simulink model "FOC_Motor"  (R2023b)
settings: Solver=FixedStepDiscrete  StartTime=0.0  StopTime=10  FixedStep=0.0001  RelTol=1e-3
undefined symbols (not defined in the file): Cos_Table, Sin_BreakPoint, Sin_Table
libraries: simulink x3
settings Model: DataDictionary=EHB_data.sldd  Creator=dell  LastModifiedBy=LQY
settings SolverCC: AlgebraicLoopSolver=TrustRegion  PositivePriorityOrder=on  AutoInsertRateTranBlk=on
settings DataIOCC: LimitDataPoints=on  SaveFormat=Structure  SignalLoggingSaveFormat=ModelDataLogs  ReturnWorkspaceOutputs=off
settings OptimizationCC: DefaultParameterBehavior=Inlined  UseDivisionForNetSlopeComputation=on  GainParamInheritBuiltInType=on  UseFloatMulNetSlope=on  InlineInvariantSignals=on  PassReuseOutputArgsAs=Individual arguments  ExpressionDepthLimit=2147483647  ZeroExternalMemoryAtStartup=off  ZeroInternalMemoryAtStartup=off  NoFixptDivByZeroProtection=on  EfficientFloat2IntCast=on  LifeSpan=1  MaxStackSize=64  EfficientTunableParamExpr=on
settings DebuggingCC: CheckSSInitialOutputMsg=off  UnderspecifiedInitializationDetection=Classic  MergeDetectMultiDrivingBlocksExec=none  SolverPrmCheckMsg=warning  ParameterOverflowMsg=none  ParameterPrecisionLossMsg=none  FcnCallInpInsideContextMsg=warning  UnconnectedInputMsg=warning  UnconnectedOutputMsg=warning  UnconnectedLineMsg=warning  AssertControl=EnableAll  StateNameClashWarn=warning  SFUnexpectedBacktrackingDiag=warning  SFNoUnconditionalDefaultTransitionDiag=warning  SFExecutionAtInitializationDiag=none  ArithmeticOperatorsInVariantConditions=warning
settings HardwareCC: ProdBitPerPointer=32  ProdBitPerSizeT=32  ProdBitPerPtrDiffT=32  ProdLargestAtomicInteger=Long  ProdLargestAtomicFloat=Double  ProdWordSize=32  ProdLongLongMode=on  ProdHWDeviceType=NXP->Cortex-M0/M0+  TargetBitPerPointer=64  TargetBitPerSizeT=64  TargetBitPerPtrDiffT=64  TargetLargestAtomicInteger=Integer  TargetLongLongMode=on  TargetIntDivRoundTo=Zero  TargetEndianess=LittleEndian  TargetWordSize=64  TargetHWDeviceType=MATLAB Host  ProdEqTarget=off
settings ModelReferenceCC: UpdateModelReferenceTargets=IfOutOfDate  EnableRefExpFcnMdlSchedulingChecks=on  PropagateSignalLabelsOutOfModel=off
settings SFSimCC: SimUseLocalCustomCode=off  MATLABDynamicMemAlloc=off  CustomCodeUndefinedFunction=UseInterfaceOnly
settings SFSimCC: SimCustomHeaderCode=|
  | #define MCU_IDLE_ST     0
  | #define MCU_INIT_ST     1
  | #define MCU_START_ST    2
  | #define MCU_RUN_ST      3
  | #define MCU_FAULT_ST    4
  | #define MCU_WAIT_ST     5
  | 
  | // MCU_IDLE_ST = 0;
  | // MCU_INIT_ST = 1;
  | // MCU_START_ST = 2;
  | // MCU_RUN_ST = 3;
  | // MCU_FAULT_ST = 4;
  | // MCU_WAIT_ST = 5;
settings RTWCC: Description=Embedded Coder  SystemTargetFile=ert.tlc  GenCodeOnly=on  TemplateMakefile=ert_default_tmf  RTWUseLocalCustomCode=off  RTWUseSimCustomCode=on  IncludeHyperlinkInReport=on
settings RTWCC: CustomHeaderCode=|
  | #define MCU_IDLE_ST     0
  | #define MCU_INIT_ST     1
  | #define MCU_START_ST    2
  | #define MCU_RUN_ST      3
  | #define MCU_FAULT_ST    4
  | #define MCU_WAIT_ST     5
  | 
  | // MCU_IDLE_ST = 0;
  | // MCU_INIT_ST = 1;
  | // MCU_START_ST = 2;
  | // MCU_RUN_ST = 3;
  | // MCU_FAULT_ST = 4;
  | // MCU_WAIT_ST = 5;
settings CodeAppCC: ForceParamTrailComments=on  IgnoreCustomStorageClasses=off  SimulinkDataObjDesc=on  CustomSymbolStrGlobalVar=rt$N$M  CustomSymbolStrType=$N$M  CustomSymbolStrFcn=$N$M$F  CustomSymbolStrMacro=$N$M  InsertBlockDesc=on  InternalIdentifier=Classic
settings ERTTargetCC: MultiwordLength=2048  IncludeMdlTerminateFcn=off  CombineSignalStateStructs=on  IncludeFileDelimiter=UseQuote  SupportAbsoluteTime=off  SupportComplex=off  SupportNonInlinedSFcns=on  InlinedParameterPlacement=NonHierarchical  ERTCustomFileTemplate=example_file_process.tlc  GlobalDataDefinition=InSeparateSourceFile  DataDefinitionFile=EHB_MOTOR_data.c  GlobalDataReference=InSeparateHeaderFile  ERTFilePackagingFormat=CompactWithDataFile  DataReferenceFile=EHB_MOTOR.h  ConvertIfToSwitch=off  SuppressUnreachableDefaultCases=off  IndentStyle=Allman  IndentSize=4  MemSecPackage=mpt
settings ConfigComp: CovMetricSettings=dw  CovSaveCumulativeToWorkspaceVar=on  CovSaveSingleToWorkspaceVar=on  CovExternalEMLEnable=off  CovSFcnEnable=off
settings SimscapeCC: SimscapeNormalizeSystem=off
settings ConfigurationSet: Description=SimMechanics 2G

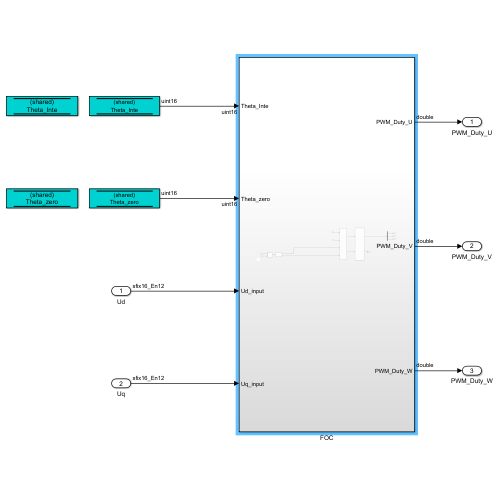
[thumbnail: Simulink's stored preview of the top-level diagram]
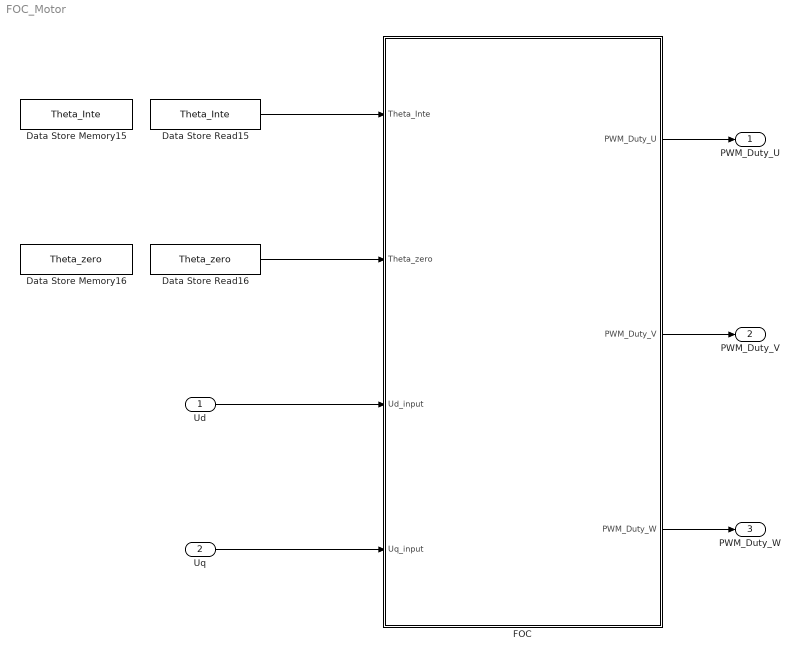
== system FOC_Motor ==
  Ud : Inport  OutDataTypeStr=fixdt(1,16,12)
  Uq : Inport  Port=2  OutDataTypeStr=fixdt(1,16,12)
  Data Store Memory15 : DataStoreMemory  DataStoreName=Theta_Inte  ReadBeforeWriteMsg=warning  WriteAfterWriteMsg=warning  WriteAfterReadMsg=warning  ShareAcrossModelInstances=on  ShowAdditionalParam=off  OutDataTypeStr=uint16
  Data Store Memory16 : DataStoreMemory  DataStoreName=Theta_zero  ReadBeforeWriteMsg=warning  WriteAfterWriteMsg=warning  WriteAfterReadMsg=warning  ShareAcrossModelInstances=on  ShowAdditionalParam=off  OutDataTypeStr=uint16
  Data Store Read15 : DataStoreRead  DataStoreName=Theta_Inte  DataStoreElements=Theta_Inte  IndexOptions=Index vector (dialog)  Indices=1  OutputSizes=1
  Data Store Read16 : DataStoreRead  DataStoreName=Theta_zero  DataStoreElements=Theta_zero  IndexOptions=Index vector (dialog)  Indices=1  OutputSizes=1
  FOC : Subsystem
  PWM_Duty_U : Outport  VectorParamsAs1DForOutWhenUnconnected=off
  PWM_Duty_V : Outport  Port=2  VectorParamsAs1DForOutWhenUnconnected=off
  PWM_Duty_W : Outport  Port=3  VectorParamsAs1DForOutWhenUnconnected=off
  wires:
  Data Store Read15/1 -> FOC/1(Theta_Inte)
  FOC/2(PWM_Duty_V) -> PWM_Duty_V/1
  FOC/1(PWM_Duty_U) -> PWM_Duty_U/1
  FOC/3(PWM_Duty_W) -> PWM_Duty_W/1
  Data Store Read16/1 -> FOC/2(Theta_zero)
  Ud/1 -> FOC/3(Ud_input)
  Uq/1 -> FOC/4(Uq_input)

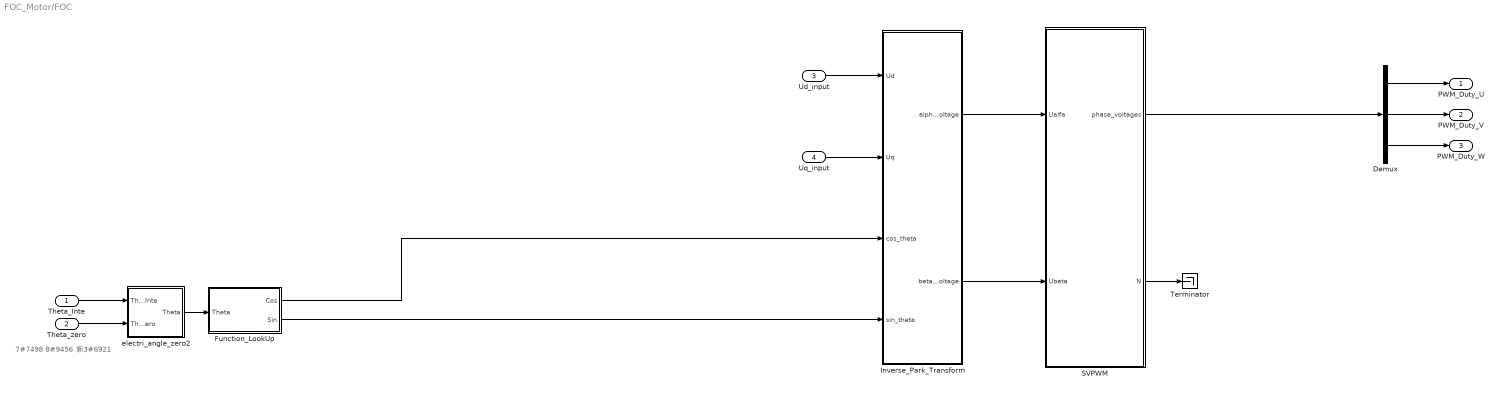
== system FOC_Motor/FOC ==
  note: 7#7498
      | 8#9456
      | 新3#6921
  Theta_Inte : Inport  OutDataTypeStr=uint16
  Theta_zero : Inport  Port=2  OutDataTypeStr=uint16
  Ud_input : Inport  Port=3
  Uq_input : Inport  Port=4
  Demux : Demux  Outputs=3
  Function_LookUp : Subsystem
  Inverse_Park_Transform : Subsystem
  SVPWM : Subsystem
  Terminator : Terminator
  electri_angle_zero2 : Subsystem
  PWM_Duty_U : Outport  VectorParamsAs1DForOutWhenUnconnected=off
  PWM_Duty_V : Outport  Port=2  VectorParamsAs1DForOutWhenUnconnected=off
  PWM_Duty_W : Outport  Port=3  VectorParamsAs1DForOutWhenUnconnected=off
  wires:
  Inverse_Park_Transform/2(beta_voltage) -> SVPWM/2(Ubeta)
  Demux/1 -> PWM_Duty_U/1
  Theta_zero/1 -> electri_angle_zero2/2(Theta_zero)
  Uq_input/1 -> Inverse_Park_Transform/2(Uq)
  Theta_Inte/1 -> electri_angle_zero2/1(Theta_Inte)
  Inverse_Park_Transform/1(alpha_voltage) -> SVPWM/1(Ualfa)
  Ud_input/1 -> Inverse_Park_Transform/1(Ud)
  SVPWM/1(phase_voltages) -> Demux/1
  Demux/3 -> PWM_Duty_W/1
  Demux/2 -> PWM_Duty_V/1
  Function_LookUp/1(Cos) -> Inverse_Park_Transform/3(cos_theta)
  Function_LookUp/2(Sin) -> Inverse_Park_Transform/4(sin_theta)
  electri_angle_zero2/1(Theta) -> Function_LookUp/1(Theta)
  SVPWM/2(N) -> Terminator/1

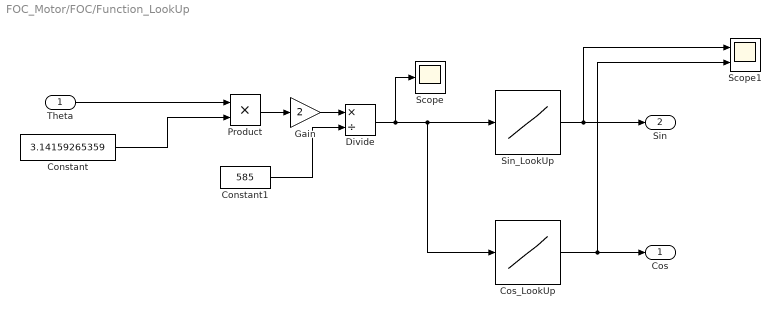
== system FOC_Motor/FOC/Function_LookUp ==
  Theta : Inport
  Constant : Constant  Value=3.14159265359
  Constant1 : Constant  Value=585
  Cos_LookUp : Lookup_n-D  NumberOfTableDimensions=1  BreakpointsForDimension1=Sin_BreakPoint  BreakpointsForDimension3=[5, 7]  BreakpointsForDimension1DataTypeStr=Inherit: Inherit from 'Breakpoint data'  Table=Cos_Table  TableDataTypeStr=Inherit: Inherit from 'Table data'  ExtrapMethod=Clip  InternalRulePriority=Speed  OutDataTypeStr=Inherit: Inherit from 'Table data'  RndMeth=Simplest  InputSameDT=off
  Divide : Product  Inputs=*/
  Gain : Gain  Gain=2
  Product : Product
  Scope : Scope
  Scope1 : Scope  NumInputPorts=2
  Sin_LookUp : Lookup_n-D  NumberOfTableDimensions=1  BreakpointsForDimension1=Sin_BreakPoint  BreakpointsForDimension3=[5, 7]  BreakpointsForDimension1DataTypeStr=Inherit: Inherit from 'Breakpoint data'  Table=Sin_Table  TableDataTypeStr=Inherit: Inherit from 'Table data'  ExtrapMethod=Clip  InternalRulePriority=Speed  OutDataTypeStr=Inherit: Inherit from 'Table data'  RndMeth=Simplest  InputSameDT=off
  Cos : Outport  VectorParamsAs1DForOutWhenUnconnected=off
  Sin : Outport  Port=2  VectorParamsAs1DForOutWhenUnconnected=off
  wires:
  Divide/1 -> Scope/1, Cos_LookUp/1, Sin_LookUp/1
  Theta/1 -> Product/1
  Cos_LookUp/1 -> Scope1/2, Cos/1
  Constant/1 -> Product/2
  Product/1 -> Gain/1
  Constant1/1 -> Divide/2
  Gain/1 -> Divide/1
  Sin_LookUp/1 -> Scope1/1, Sin/1

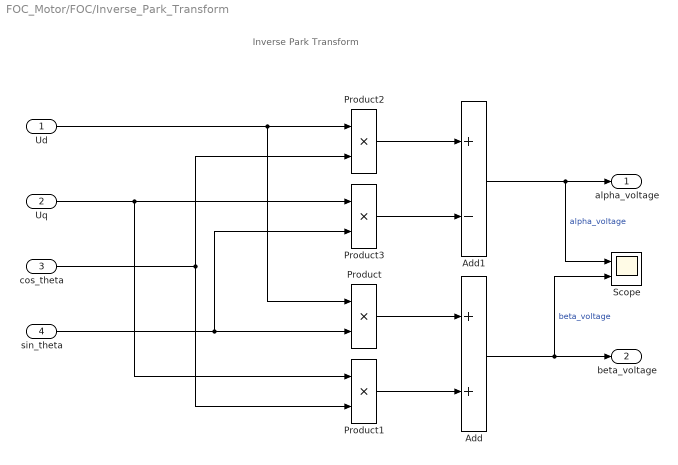
== system FOC_Motor/FOC/Inverse_Park_Transform ==
  note: Inverse Park Transform
  Ud : Inport
  Uq : Inport  Port=2
  cos_theta : Inport  Port=3
  sin_theta : Inport  Port=4
  Add : Sum  OutDataTypeStr=fixdt(1,16,12)
  Add1 : Sum  Inputs=+-  OutDataTypeStr=fixdt(1,16,12)
  Product{,1..3} (4 alike) : Product  OutDataTypeStr=fixdt(1,16,12)  RndMeth=Zero
  Scope : Scope  NumInputPorts=2
  alpha_voltage : Outport  VectorParamsAs1DForOutWhenUnconnected=off
  beta_voltage : Outport  Port=2  VectorParamsAs1DForOutWhenUnconnected=off
  wires:
  Product/1 -> Add/1
  Product1/1 -> Add/2
  Add/1 -> Scope/2, beta_voltage/1  "beta_voltage"
  Product2/1 -> Add1/1
  Product3/1 -> Add1/2
  Add1/1 -> Scope/1, alpha_voltage/1  "alpha_voltage"
  Ud/1 -> Product/1, Product2/1
  sin_theta/1 -> Product/2, Product3/2
  cos_theta/1 -> Product1/2, Product2/2
  Uq/1 -> Product1/1, Product3/1

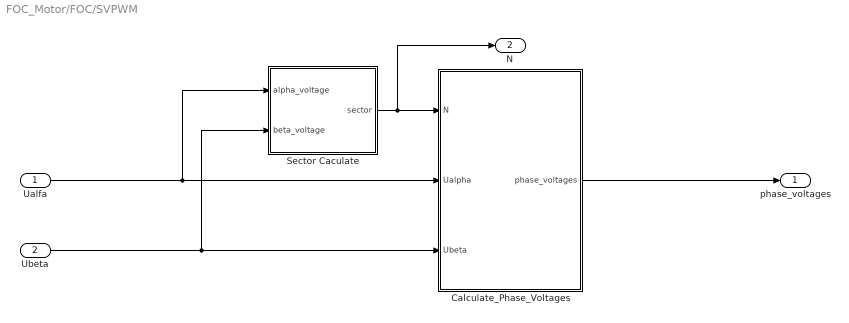
== system FOC_Motor/FOC/SVPWM ==
  Ualfa : Inport  OutDataTypeStr=fixdt(1,16,12)
  Ubeta : Inport  Port=2
  Calculate_Phase_Voltages : Subsystem
  Sector Caculate : Subsystem
  phase_voltages : Outport  VectorParamsAs1DForOutWhenUnconnected=off
  N : Outport  Port=2  VectorParamsAs1DForOutWhenUnconnected=off
  wires:
  Ualfa/1 -> Sector Caculate/1(alpha_voltage), Calculate_Phase_Voltages/2(Ualpha)
  Ubeta/1 -> Calculate_Phase_Voltages/3(Ubeta), Sector Caculate/2(beta_voltage)
  Calculate_Phase_Voltages/1(phase_voltages) -> phase_voltages/1
  Sector Caculate/1(sector) -> N/1, Calculate_Phase_Voltages/1(N)

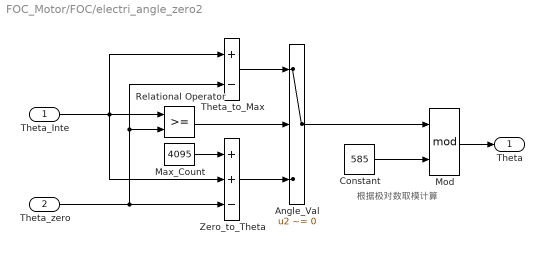
== system FOC_Motor/FOC/electri_angle_zero2 ==
  note: 根据极对数取模计算
  Theta_Inte : Inport
  Theta_zero : Inport  Port=2  OutDataTypeStr=uint16
  Angle_Val : Switch  Criteria=u2 ~= 0  Threshold=3032  OutDataTypeStr=uint16  SaturateOnIntegerOverflow=off  InputSameDT=off
  Constant : Constant  Value=585  OutDataTypeStr=uint16
  Max_Count : Constant  Value=4095  OutDataTypeStr=uint16
  Mod : Math  Operator=mod  SignedPower=on
  Relational Operator : RelationalOperator  OutDataTypeStr=boolean  InputSameDT=off
  Theta_to_Max : Sum  Inputs=+-  OutDataTypeStr=uint16
  Zero_to_Theta : Sum  Inputs=++-  OutDataTypeStr=uint16
  Theta : Outport  VectorParamsAs1DForOutWhenUnconnected=off
  wires:
  Max_Count/1 -> Zero_to_Theta/1
  Theta_zero/1 -> Zero_to_Theta/3, Theta_to_Max/2, Relational Operator/2
  Theta_Inte/1 -> Zero_to_Theta/2, Theta_to_Max/1, Relational Operator/1
  Zero_to_Theta/1 -> Angle_Val/3
  Angle_Val/1 -> Mod/1
  Theta_to_Max/1 -> Angle_Val/1
  Relational Operator/1 -> Angle_Val/2
  Mod/1 -> Theta/1
  Constant/1 -> Mod/2

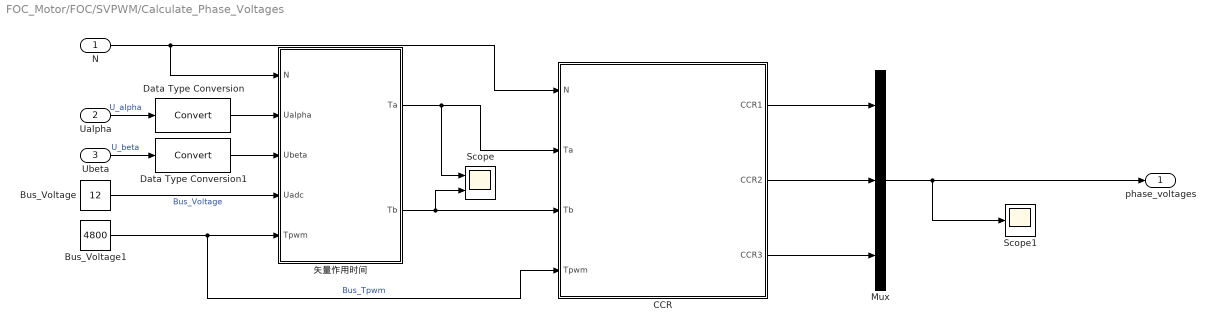
== system FOC_Motor/FOC/SVPWM/Calculate_Phase_Voltages ==
  N : Inport  OutDataTypeStr=uint8
  Ualpha : Inport  Port=2
  Ubeta : Inport  Port=3
  Bus_Voltage : Constant  Value=12  OutDataTypeStr=double
  Bus_Voltage1 : Constant  Value=4800  OutDataTypeStr=double
  CCR : MATLAB Function  TreatAsAtomicUnit=on
  Data Type Conversion : DataTypeConversion  SaturateOnIntegerOverflow=off  RndMeth=Floor
  Data Type Conversion1 : DataTypeConversion  SaturateOnIntegerOverflow=off  RndMeth=Floor
  Mux : Mux  Inputs=3
  Scope : Scope  NumInputPorts=2
  Scope1 : Scope
  矢量作用时间 : MATLAB Function  TreatAsAtomicUnit=on
  phase_voltages : Outport  VectorParamsAs1DForOutWhenUnconnected=off
  wires:
  Ualpha/1 -> Data Type Conversion/1  "U_alpha"
  Ubeta/1 -> Data Type Conversion1/1  "U_beta"
  Bus_Voltage/1 -> 矢量作用时间/4(Uadc)  "Bus_Voltage"
  N/1 -> 矢量作用时间/1(N), CCR/1(N)
  Bus_Voltage1/1 -> CCR/4(Tpwm), 矢量作用时间/5(Tpwm)  "Bus_Tpwm"
  矢量作用时间/1(Ta) -> Scope/1, CCR/2(Ta)
  矢量作用时间/2(Tb) -> Scope/2, CCR/3(Tb)
  CCR/1(CCR1) -> Mux/1
  CCR/2(CCR2) -> Mux/2
  CCR/3(CCR3) -> Mux/3
  Mux/1 -> Scope1/1, phase_voltages/1
  Data Type Conversion/1 -> 矢量作用时间/2(Ualpha)
  Data Type Conversion1/1 -> 矢量作用时间/3(Ubeta)

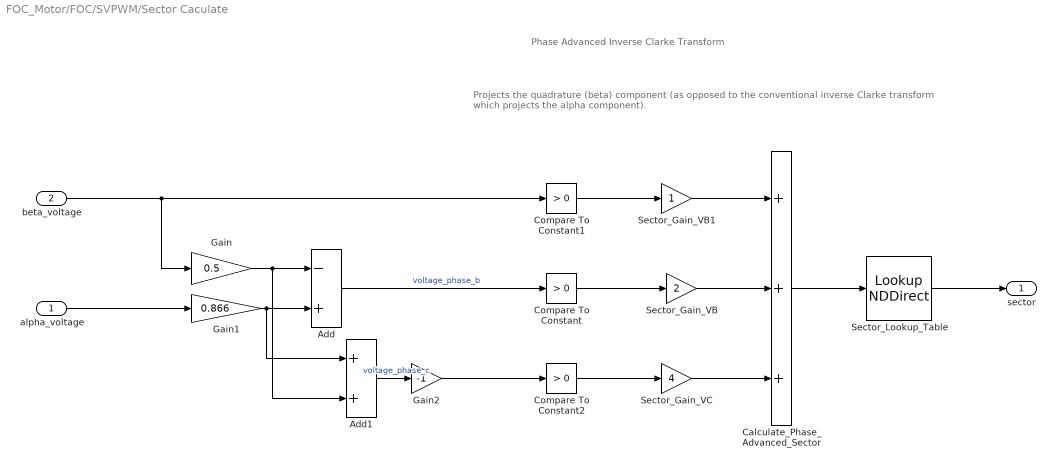
== system FOC_Motor/FOC/SVPWM/Sector Caculate ==
  note: Phase Advanced Inverse Clarke Transform
  note: Projects the quadrature (beta) component (as opposed to the conventional inverse Clarke transform
      | which projects the alpha component).
  alpha_voltage : Inport
  beta_voltage : Inport  Port=2
  Add : Sum  Inputs=-+
  Add1 : Sum
  Calculate_Phase_Advanced_Sector : Sum  Inputs=+++  OutDataTypeStr=uint8  AccumDataTypeStr=uint8
  Compare To Constant : simulink/Logic and Bit Operations/Compare To Constant  relop=>  const=0  OutDataTypeStr=boolean
  Compare To Constant1 : simulink/Logic and Bit Operations/Compare To Constant  relop=>  const=0  OutDataTypeStr=boolean
  Compare To Constant2 : simulink/Logic and Bit Operations/Compare To Constant  relop=>  const=0  OutDataTypeStr=boolean
  Gain : Gain  Gain=0.5  OutDataTypeStr=Inherit: Same as input
  Gain1 : Gain  Gain=0.866  OutDataTypeStr=Inherit: Same as input
  Gain2 : Gain  Gain=-1
  Sector_Gain_VB : Gain  Gain=2  ParamDataTypeStr=int16  OutDataTypeStr=uint8
  Sector_Gain_VB1 : Gain  ParamDataTypeStr=int16  OutDataTypeStr=uint8
  Sector_Gain_VC : Gain  Gain=4  ParamDataTypeStr=int16  OutDataTypeStr=uint8
  Sector_Lookup_Table : LookupNDDirect  NumberOfTableDimensions=1  Table=[2,2,6,1,4,3,5]  TableDataTypeStr=uint8
      settings: AttributesFormatString=-------------------------------\nTable: %<Table>
  sector : Outport  VectorParamsAs1DForOutWhenUnconnected=off
  wires:
  Sector_Gain_VC/1 -> Calculate_Phase_Advanced_Sector/3
  alpha_voltage/1 -> Gain1/1
  Calculate_Phase_Advanced_Sector/1 -> Sector_Lookup_Table/1
  Sector_Lookup_Table/1 -> sector/1
  Compare To Constant1/1 -> Sector_Gain_VB1/1
  beta_voltage/1 -> Compare To Constant1/1, Gain/1
  Add1/1 -> Gain2/1  "voltage_phase_c"
  Compare To Constant2/1 -> Sector_Gain_VC/1
  Compare To Constant/1 -> Sector_Gain_VB/1
  Sector_Gain_VB/1 -> Calculate_Phase_Advanced_Sector/2
  Gain/1 -> Add/1, Add1/2
  Add/1 -> Compare To Constant/1  "voltage_phase_b"
  Sector_Gain_VB1/1 -> Calculate_Phase_Advanced_Sector/1
  Gain1/1 -> Add1/1, Add/2
  Gain2/1 -> Compare To Constant2/1

== matlab function FOC_Motor/FOC/SVPWM/Calculate_Phase_Voltages/CCR ==
  data: N input; CCR1 output; Ta input; Tb input; Tpwm input; CCR2 output; CCR3 output
function [CCR1,CCR2,CCR3] = fcn(N,Ta,Tb,Tpwm)

CCR1=double(0);
CCR2=double(0);
CCR3=double(0);

Temp=Ta+Tb;
if(Temp>Tpwm)
    Ta=Ta/Temp*Tpwm;
    Tb=Tb/Temp*Tpwm;
end
T0 = Tpwm - Ta - Tb;

value1=(Ta+Tb+T0/2)/2;
value2=(Tb+T0/2)/2;
value3=(T0/2)/2;

switch(N)
    case 1
        CCR1=value1;
        CCR2=value2;
        CCR3=value3;
    case 2
        CCR1=value2;
        CCR2=value1;
        CCR3=value3;
    case 3
        CCR1=value3;
        CCR2=value1;
        CCR3=value2;
    case 4
        CCR1=value3;
        CCR2=value2;
        CCR3=value1;
    case 5
        CCR1=value2;
        CCR2=value3;
        CCR3=value1;
    case 6
        CCR1=value1;
        CCR2=value3;
        CCR3=value2;
end

== matlab function FOC_Motor/FOC/SVPWM/Calculate_Phase_Voltages/矢量作用时间 ==
  data: N input; Ta output; Ualpha input; Ubeta input; Uadc input; Tpwm input; Tb output
function [Ta,Tb] = fcn(N,Ualpha,Ubeta,Uadc,Tpwm)

Ta=double(0);
Tb=double(0);
X=(sqrt(3)*Tpwm)/Uadc*Ubeta;            %系数1 
Y=(sqrt(3)*Tpwm)/Uadc*((sqrt(3)/2)*Ualpha-(1/2)*Ubeta);  %系数2
Z=(sqrt(3)*Tpwm)/Uadc*(-(sqrt(3)/2)*Ualpha-(1/2)*Ubeta);   %系数3
    
if(N==1)   %第一扇区
   Ta=Y;
   Tb=X;
end
if(N==2)   %第二扇区
   Ta=-Y;
   Tb=-Z;
end
if(N==3)   %第三扇区
   Ta=X;
   Tb=Z;
end
if(N==4)   %第四扇区
   Ta=-X;
   Tb=-Y;
end
if(N==5)   %第五扇区
   Ta=Z;
   Tb=Y;
end
if(N==6)   %第六扇区
   Ta=-Z;
   Tb=-X;
end
